simulink model "GEWT_MSC_parthelper2"  (R2015b)
settings: Solver=VariableStepAuto  StartTime=0.0  StopTime=10.0  RelTol=1e-3
values from neighbouring files (symbols this model uses):
  drivefreq = 30e3    (= 30000)    [GEWT.m]
  fluxlinkage = 1.5    [GEWT.m]
  gear = 117.4    [GEWT.m]
  Jtotal = Jgen+Jtur/(gear^2)    (= 1143.20731116)    [GEWT.m]
  Ld = 2.48e-4    (= 0.000248)    [GEWT.m]
  Lq = 2.92e-4    (= 0.000292)    [GEWT.m]
  p = 1.225    [GEWT.m]
  Prated = 2750000    [GEWT.m]
  R = 51.5    [GEWT.m]
  Rs = 0.7305e-3    (= 0.0007305)    [GEWT.m]
  Ts = 2E-6    (= 2e-06)    [GEWT.m]
  windspeed = 10    [GEWT.m]
libraries: powerlib x7, powerlib_meascontrol x5, simulink x3
settings Model: Creator=Eren  LastModifiedBy=Eren

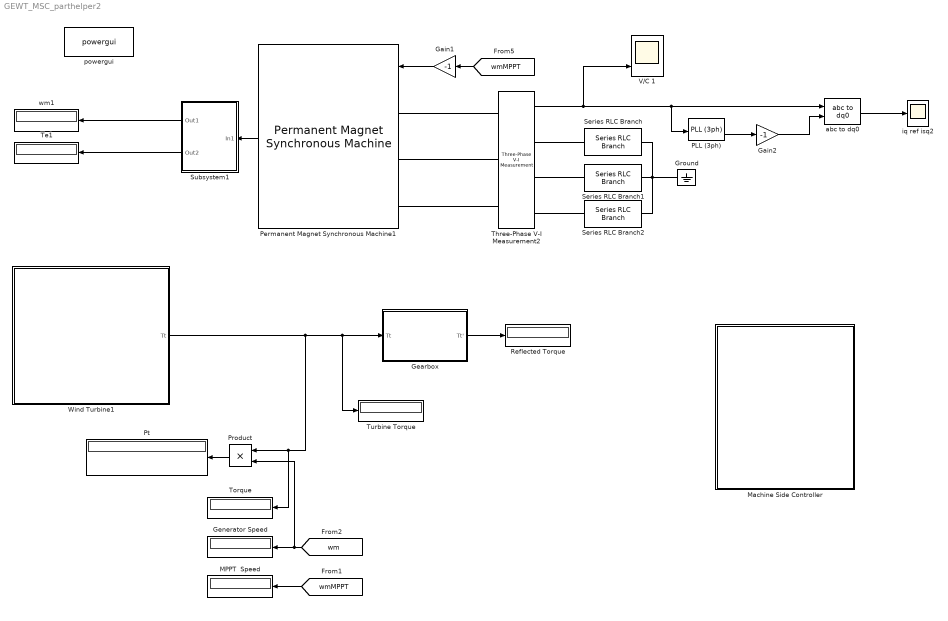
== system GEWT_MSC_parthelper2 ==
  Gain1 : Gain  Gain=-1
  Gain2 : Gain  Gain=-1
  Gearbox : Subsystem
  Generator Speed : Display
  Ground : powerlib/Elements/Ground  LConnTagsString=a
  MPPT  Speed : Display
  "Machine Side Controller " : Subsystem
  PLL (3ph) : powerlib_meascontrol/PLL/PLL (3ph)  Fmin=45  Par_Init=[0, 50]  ParK=[180, 3200, 1]  TcD=1e-4  MaxRateChangeFreq=12  FilterCutOffFreq=25  Ts=Ts  AGC=on
  Permanent Magnet Synchronous Machine1 : powerlib/Machines/Permanent Magnet Synchronous Machine  NbPhases=3  FluxDistribution=Sinusoidal  RotorType=Salient-pole  MechanicalLoad=Speed w  PresetModel=No  ShowDetailedParameters=on  MeasurementBus=off  Resistance=Rs  Inductance=8.5e-3  dqInductances=[Ld,Lq]  La=0.001764  MachineConstant=Voltage Constant (V_peak L-L / krpm)  Flux=1.7933  VoltageCst=650.538  TorqueCst=5.3799  Flat=120  Mechanical=[Jtotal 1.349e-05 4 0]  PolePairs=2  InitialConditions=[-168.8,0, 0,0]  InitialConditions5ph=[0 0 0 0 0 0]  TsPowergui=0  TsBlock=-1  RefAngle=90 degrees behind phase A axis (modified Park)
  Product : Product
  Pt : Display
  Reflected Torque : Display
  Series RLC Branch : powerlib/Elements/Series RLC Branch  LConnTagsString=__new0  RConnTagsString=__new0  BranchType=R  Resistance=1  Inductance=1e-3  SetiL0=off  InitialCurrent=0  Capacitance=1e-6  Setx0=off  InitialVoltage=0  Measurements=None
  Series RLC Branch1 : powerlib/Elements/Series RLC Branch  LConnTagsString=__new0  RConnTagsString=__new0  BranchType=R  Resistance=1  Inductance=1e-3  SetiL0=off  InitialCurrent=0  Capacitance=1e-6  Setx0=off  InitialVoltage=0  Measurements=None
  Series RLC Branch2 : powerlib/Elements/Series RLC Branch  LConnTagsString=__new0  RConnTagsString=__new0  BranchType=R  Resistance=1  Inductance=1e-3  SetiL0=off  InitialCurrent=0  Capacitance=1e-6  Setx0=off  InitialVoltage=0  Measurements=None
  Subsystem1 : Subsystem
  Te1 : Display
  Three-Phase V-I Measurement2 : powerlib/Measurements/Three-Phase V-I Measurement  VoltageMeasurement=phase-to-ground  SetLabelV=off  LabelV=Vsabc  Vpu=off  VpuLL=off  CurrentMeasurement=yes  SetLabelI=on  LabelI=Isabc  Ipu=off  Pbase=10e6  Vbase=690  OutputType=Complex  PhasorSimulation=off  PSBequivalent=0
  Torque : Display
  Turbine Torque : Display
  V/C 1 : Scope  NumInputPorts=2
  Wind Turbine1 : Subsystem
  abc to dq0 : powerlib_meascontrol/Transformations/abc to dq0  Alignment=90 degrees behind phase A axis
  iq ref isq2 : Scope
  powergui : powerlib/powergui  Priority=2  SimulationMode=Discrete  SolverType=Tustin  SampleTime=Ts  frequency=60  SPID=off  DisableSnubberDevices=off  DisableRonSwitches=off  DisableVfSwitches=off  SwTol=0  DisplayEquations=off  Interpol=off  ExternalGateDelay=off  methode=off  Ts=0  FunctionMessages=off  echomessages=off  HookPort=off  EnableUseOfTLC=off  x0status=blocks  frequencyindice=0  Pbase=100e6  ErrMax=1e-4  Iterations=50  UnitsV=kV  UnitsW=MW  buscounter=0  RestoreLinks=warning  ResistiveCurrentMeasurement=off  Frange=[0:2:500]  Ylog=off  Xlog=on  ShowGrid=off  save=off  variable=ZData  structure=0  ZoomFFT=on  StartTime=0.0  cycles=1  DisplayStyle=1  fundamental=60  FreqAxis=off  MaxFrequency=1000  frequencyindicesteady=1  RmsSteady=1  display=off
  wm1 : Display
  wires:
  Permanent Magnet Synchronous Machine1/1 -> Subsystem1/1(In1)
  Subsystem1/1(Out1) -> wm1/1
  Subsystem1/2(Out2) -> Te1/1
  [wmMPPT] -> Gain1/1
  Gain1/1 -> Permanent Magnet Synchronous Machine1/1
  Three-Phase V-I Measurement2/1 -> PLL (3ph)/1, abc to dq0/1, V/C 1/2
  [wm] -> Generator Speed/1, Product/2
  Product/1 -> Pt/1
  Wind Turbine1/1(Tt) -> Turbine Torque/1, Gearbox/1(Tt), Product/1, Torque/1
  Gearbox/1(Tt') -> Reflected Torque/1
  PLL (3ph)/2 -> Gain2/1
  abc to dq0/1 -> iq ref isq2/1
  Gain2/1 -> abc to dq0/2
  [wmMPPT] -> MPPT  Speed/1
  connections:
  Permanent Magnet Synchronous Machine1/LConn2 -- Three-Phase V-I Measurement2/LConn2
  Permanent Magnet Synchronous Machine1/LConn1 -- Three-Phase V-I Measurement2/LConn1
  Permanent Magnet Synchronous Machine1/LConn3 -- Three-Phase V-I Measurement2/LConn3
  Series RLC Branch2/LConn1 -- Three-Phase V-I Measurement2/RConn3
  Series RLC Branch1/LConn1 -- Three-Phase V-I Measurement2/RConn2
  Series RLC Branch/LConn1 -- Three-Phase V-I Measurement2/RConn1
  Series RLC Branch/RConn1 -- Ground/LConn1 -- Series RLC Branch2/RConn1 -- Series RLC Branch1/RConn1

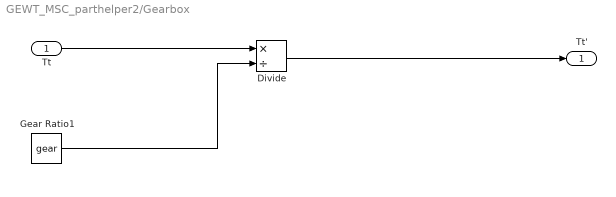
== system GEWT_MSC_parthelper2/Gearbox ==
  Tt : Inport
  Divide : Product  Inputs=*/
  Gear Ratio1 : Constant  Value=gear
  Tt' : Outport
  wires:
  Gear Ratio1/1 -> Divide/2
  Tt/1 -> Divide/1
  Divide/1 -> Tt'/1

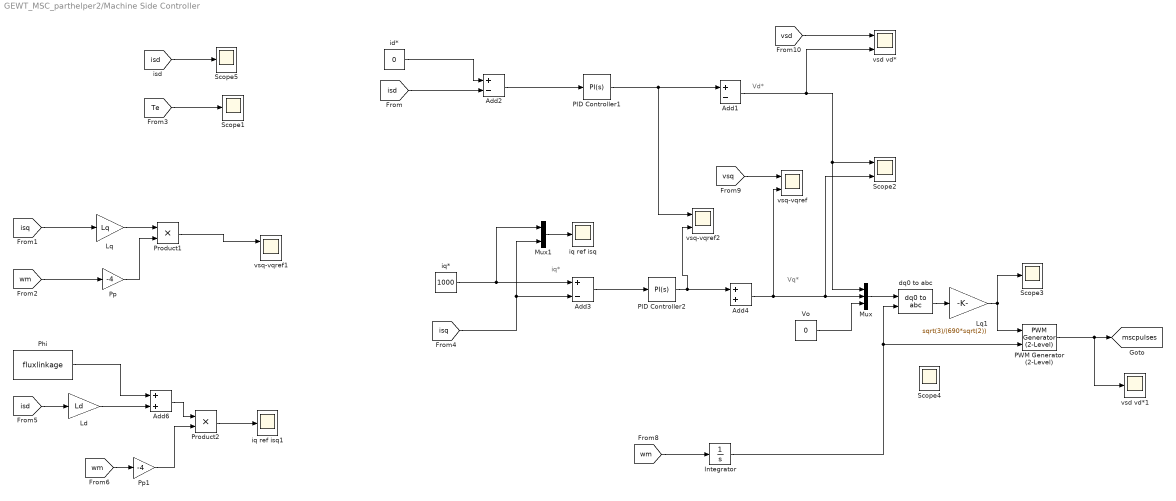
== system GEWT_MSC_parthelper2/Machine Side Controller  ==
  note: iq*
  note: Vq*
  note: Vd*
  Add1 : Sum  Inputs=+-
  Add2 : Sum  Inputs=+-
  Add3 : Sum  Inputs=+-
  Add4 : Sum
  Add6 : Sum
  Integrator : Integrator
  Ld : Gain  Gain=Ld
  Lq : Gain  Gain=Lq
  Lq1 : Gain  Gain=sqrt(3)/(690*sqrt(2))
  Mux : Mux  Inputs=3
  Mux1 : Mux  Inputs=2
  PID Controller1 : simulink/Continuous/PID Controller  Controller=PI  TimeDomain=Continuous-time  SampleTime=-1  IntegratorMethod=Forward Euler  FilterMethod=Forward Euler  Form=Ideal  UseFilter=on  ControllerParametersSource=internal  P=0.0001  I=0.00001  D=0  N=100  InitialConditionSource=internal  InitialConditionForIntegrator=0  InitialConditionForFilter=0  ExternalReset=none  LimitOutput=on  UpperSaturationLimit=2*690  LowerSaturationLimit=-2*690  LinearizeAsGain=on  AntiWindupMode=none  Kb=1  TrackingMode=off  Kt=1  PParamMin=[]  PParamMax=[]  IParamMin=[]  IParamMax=[]  DParamMin=[]  DParamMax=[]  NParamMin=[]  NParamMax=[]  KbParamMin=[]  KbParamMax=[]  KtParamMin=[]  KtParamMax=[]  POutMin=[]  POutMax=[]  IOutMin=[]  IOutMax=[]  DOutMin=[]  DOutMax=[]  NOutMin=[]  NOutMax=[]  KbOutMin=[]  KbOutMax=[]  KtOutMin=[]  KtOutMax=[]  IntegratorOutMin=[]  IntegratorOutMax=[]  FilterOutMin=[]  FilterOutMax=[]  SumOutMin=[]  SumOutMax=[]  SumI1OutMin=[]  SumI1OutMax=[]  SumI2OutMin=[]  SumI2OutMax=[]  SumI3OutMin=[]  SumI3OutMax=[]  SumDOutMin=[]  SumDOutMax=[]  SaturationOutMin=[]  SaturationOutMax=[]  IntegratorContinuousStateAttributes=''  IntegratorStateMustResolveToSignalObject=off  IntegratorRTWStateStorageClass=Auto  FilterContinuousStateAttributes=''  FilterStateMustResolveToSignalObject=off  FilterRTWStateStorageClass=Auto  DifferentiatorICPrevScaledInput=0  DifferentiatorOutMin=[]  DifferentiatorOutMax=[]
  PID Controller2 : simulink/Continuous/PID Controller  Controller=PI  TimeDomain=Continuous-time  SampleTime=-1  IntegratorMethod=Forward Euler  FilterMethod=Forward Euler  Form=Ideal  UseFilter=on  ControllerParametersSource=internal  P=0.0001  I=0.00001  D=0  N=100  InitialConditionSource=internal  InitialConditionForIntegrator=0  InitialConditionForFilter=0  ExternalReset=none  LimitOutput=on  UpperSaturationLimit=2*690  LowerSaturationLimit=-2*690  LinearizeAsGain=on  AntiWindupMode=none  Kb=1  TrackingMode=off  Kt=1  PParamMin=[]  PParamMax=[]  IParamMin=[]  IParamMax=[]  DParamMin=[]  DParamMax=[]  NParamMin=[]  NParamMax=[]  KbParamMin=[]  KbParamMax=[]  KtParamMin=[]  KtParamMax=[]  POutMin=[]  POutMax=[]  IOutMin=[]  IOutMax=[]  DOutMin=[]  DOutMax=[]  NOutMin=[]  NOutMax=[]  KbOutMin=[]  KbOutMax=[]  KtOutMin=[]  KtOutMax=[]  IntegratorOutMin=[]  IntegratorOutMax=[]  FilterOutMin=[]  FilterOutMax=[]  SumOutMin=[]  SumOutMax=[]  SumI1OutMin=[]  SumI1OutMax=[]  SumI2OutMin=[]  SumI2OutMax=[]  SumI3OutMin=[]  SumI3OutMax=[]  SumDOutMin=[]  SumDOutMax=[]  SaturationOutMin=[]  SaturationOutMax=[]  IntegratorContinuousStateAttributes=''  IntegratorStateMustResolveToSignalObject=off  IntegratorRTWStateStorageClass=Auto  FilterContinuousStateAttributes=''  FilterStateMustResolveToSignalObject=off  FilterRTWStateStorageClass=Auto  DifferentiatorICPrevScaledInput=0  DifferentiatorOutMin=[]  DifferentiatorOutMax=[]
  PWM Generator (2-Level) : powerlib_meascontrol/Pulse & Signal Generators/PWM Generator (2-Level)  ModulatorType=Three-phase bridge (6 pulses)  ModulatorMode=Synchronized  Fc=drivefreq  Pc=90  nF=drivefreq/50  MinMax="[ -1  1 ]"  SamplingTechnique=Natural  ModulatingSignals=off  m=0.8  Freq=60  Phase=0  Ts=Ts  ShowCarrierOutport=off
  Phi : Constant  Value=fluxlinkage
  Pp : Gain  Gain=-4
  Pp1 : Gain  Gain=-4
  Product1 : Product
  Product2 : Product
  Scope{1,3..5} (4 alike) : Scope
  Scope2 : Scope  NumInputPorts=2
  Vo : Constant  Value=0
  dq0 to abc : powerlib_meascontrol/Transformations/dq0 to abc  Alignment=90 degrees behind phase A axis
  id* : Constant  Value=0
  iq ref isq : Scope
  iq ref isq1 : Scope
  iq* : Constant  Value=1000
  vsd vd* : Scope  NumInputPorts=2
  vsd vd*1 : Scope
  vsq-vqref : Scope  NumInputPorts=2
  vsq-vqref1 : Scope  NumInputPorts=2
  vsq-vqref2 : Scope  NumInputPorts=2
  tag scope: mscpulses=global
  wires:
  dq0 to abc/1 -> Lq1/1
  Mux/1 -> dq0 to abc/1
  id*/1 -> Add2/1
  Vo/1 -> Mux/3
  [isq] -> Add3/2, Mux1/2
  [wm] -> Pp1/1
  Add3/1 -> PID Controller2/1
  Add2/1 -> PID Controller1/1
  Pp1/1 -> Product2/2
  Ld/1 -> Add6/2
  [isd] -> Add2/2
  Lq/1 -> Product1/1
  Phi/1 -> Add6/1
  PID Controller1/1 -> vsq-vqref2/1, Add1/1
  Add6/1 -> Product2/1
  Pp/1 -> Product1/2
  [isd] -> Ld/1
  [wm] -> Pp/1
  PID Controller2/1 -> vsq-vqref2/2, Add4/1
  [isq] -> Lq/1
  [vsq] -> vsq-vqref/1
  [vsd] -> vsd vd*/1
  Mux1/1 -> iq ref isq/1
  Product1/1 -> vsq-vqref1/1
  [isd] -> Scope5/1
  [Te] -> Scope1/1
  PWM Generator (2-Level)/1 -> [mscpulses], vsd vd*1/1
  Add1/1 -> Scope2/1, Mux/1, vsd vd*/2
  Add4/1 -> Mux/2, Scope2/2, vsq-vqref/2
  iq*/1 -> Add3/1, Mux1/1
  Product2/1 -> iq ref isq1/1
  Lq1/1 -> PWM Generator (2-Level)/1, Scope3/1
  [wm] -> Integrator/1
  Integrator/1 -> PWM Generator (2-Level)/2, dq0 to abc/2

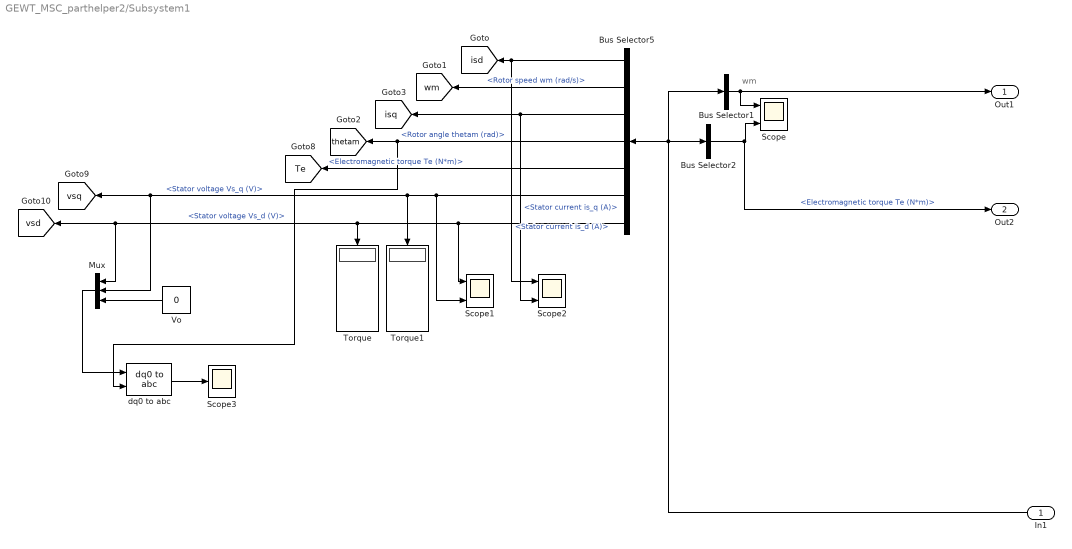
== system GEWT_MSC_parthelper2/Subsystem1 ==
  note: wm
  In1 : Inport
  Bus Selector1 : BusSelector  OutputSignals=Rotor speed wm (rad/s)  OutputAsBus=on
  Bus Selector2 : BusSelector  OutputSignals=Electromagnetic torque Te (N*m)
  Bus Selector5 : BusSelector  OutputSignals=Stator current is_d (A),Rotor speed wm (rad/s),Stator current is_q (A),Rotor angle thetam (rad),Electromagnetic torque Te (N*m),Stator voltage Vs_q (V),Stator voltage Vs_d (V)
  Mux : Mux  Inputs=3
  Scope : Scope  NumInputPorts=2
  Scope1 : Scope  NumInputPorts=2
  Scope2 : Scope  NumInputPorts=2
  Scope3 : Scope
  Torque : Display
  Torque1 : Display
  Vo : Constant  Value=0
  dq0 to abc : powerlib_meascontrol/Transformations/dq0 to abc  Alignment=90 degrees behind phase A axis
  Out1 : Outport
  Out2 : Outport  Port=2
  tag scope: Te=global, isd=global, isq=global, thetam=global, vsd=global, vsq=global, wm=global
  wires:
  Bus Selector1/1 -> Out1/1, Scope/1
  In1/1 -> Bus Selector5/1, Bus Selector1/1, Bus Selector2/1
  Bus Selector5/1 -> Scope2/1, [isd]  "<Stator current is_d (A)>"
  Bus Selector2/1 -> Out2/1, Scope/2  "<Electromagnetic torque Te (N*m)>"
  Bus Selector5/3 -> Scope2/2, [isq]  "<Stator current is_q (A)>"
  Bus Selector5/4 -> dq0 to abc/2, [thetam]  "<Rotor angle thetam (rad)>"
  Bus Selector5/5 -> [Te]  "<Electromagnetic torque Te (N*m)>"
  Bus Selector5/6 -> Scope1/2, Mux/2, [vsq], Torque1/1  "<Stator voltage Vs_q (V)>"
  Bus Selector5/7 -> Scope1/1, Mux/1, [vsd], Torque/1  "<Stator voltage Vs_d (V)>"
  Bus Selector5/2 -> [wm]  "<Rotor speed wm (rad/s)>"
  Vo/1 -> Mux/3
  Mux/1 -> dq0 to abc/1
  dq0 to abc/1 -> Scope3/1

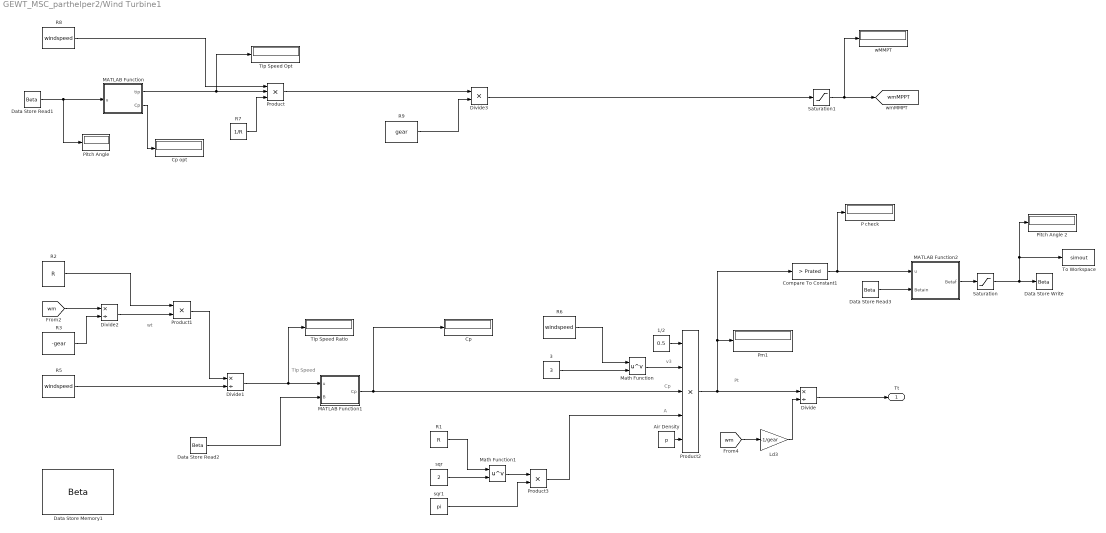
== system GEWT_MSC_parthelper2/Wind Turbine1 ==
  note: Pt
  note: v3
  note: Cp
  note: A
  note: wt
  note: Tip Speed
  1/2 : Constant  Value=0.5
  3 : Constant  Value=3
  Air Density : Constant  Value=p
  Compare To Constant1 : simulink/Logic and Bit Operations/Compare To Constant  relop=>  const=Prated  OutDataTypeStr=boolean
  Cp : Display
  Cp opt : Display
  Data Store Memory1 : DataStoreMemory  DataStoreName=Beta  ReadBeforeWriteMsg=warning  WriteAfterWriteMsg=warning  WriteAfterReadMsg=warning  OutMin=[0]  OutMax=[90]
  Data Store Read1 : DataStoreRead  DataStoreName=Beta  SampleTime=Ts
  Data Store Read2 : DataStoreRead  DataStoreName=Beta  SampleTime=Ts
  Data Store Read3 : DataStoreRead  DataStoreName=Beta  SampleTime=Ts
  Data Store Write : DataStoreWrite  DataStoreName=Beta
  Divide : Product  Inputs=*/
  Divide1 : Product  Inputs=*/
  Divide2 : Product  Inputs=*/
  Divide3 : Product  Inputs=**
  Ld3 : Gain  Gain=-1/gear
  MATLAB Function : MATLAB Function  TreatAsAtomicUnit=on
  MATLAB Function1 : MATLAB Function  TreatAsAtomicUnit=on
  MATLAB Function2 : MATLAB Function  TreatAsAtomicUnit=on
  Math Function : Math  Operator=pow  SaturateOnIntegerOverflow=on
  Math Function1 : Math  Operator=pow  SaturateOnIntegerOverflow=on
  P check : Display
  "Pitch Angle " : Display
  Pitch Angle 2 : Display
  Pm1 : Display
  Product : Product  Inputs=3
  Product1 : Product
  Product2 : Product  Inputs=5
  Product3 : Product
  R1 : Constant  Value=R
  R2 : Constant  Value=R
  R3 : Constant  Value=-gear
  R5 : Constant  Value=windspeed
  R6 : Constant  Value=windspeed
  R7 : Constant  Value=1/R
  R8 : Constant  Value=windspeed
  R9 : Constant  Value=gear
  Saturation : Saturate  UpperLimit=90  LowerLimit=0
  Saturation1 : Saturate  UpperLimit=181.68  LowerLimit=0
  "Tip Speed Opt " : Display
  "Tip Speed Ratio " : Display
  To Workspace : ToWorkspace  VariableName=simout  SaveFormat=Timeseries  SampleTime=-1
  sqr : Constant  Value=2
  sqr1 : Constant  Value=pi
  "wMMPT " : Display
  Tt : Outport
  tag scope: wmMPPT=global
  wires:
  Air Density/1 -> Product2/5
  1/2/1 -> Product2/1
  Product3/1 -> Product2/4
  Math Function1/1 -> Product3/1
  sqr1/1 -> Product3/2
  [wm] -> Ld3/1
  Math Function/1 -> Product2/2
  sqr/1 -> Math Function1/2
  R1/1 -> Math Function1/1
  Divide/1 -> Tt/1
  Product2/1 -> Divide/1, Compare To Constant1/1, Pm1/1
  3/1 -> Math Function/2
  R2/1 -> Product1/1
  [wm] -> Divide2/1
  Product1/1 -> Divide1/1
  R5/1 -> Divide1/2
  Divide1/1 -> MATLAB Function1/1(u), "Tip Speed Ratio "/1
  Divide2/1 -> Product1/2
  Ld3/1 -> Divide/2
  MATLAB Function1/1(Cp) -> Product2/3, Cp/1
  R3/1 -> Divide2/2
  R6/1 -> Math Function/1
  MATLAB Function/1(tip) -> "Tip Speed Opt "/1, Product/2
  R7/1 -> Product/3
  R8/1 -> Product/1
  Product/1 -> Divide3/1
  R9/1 -> Divide3/2
  MATLAB Function/2(Cp) -> Cp opt/1
  Divide3/1 -> Saturation1/1
  Data Store Read3/1 -> MATLAB Function2/2(Betain)
  Data Store Read2/1 -> MATLAB Function1/2(B)
  Data Store Read1/1 -> "Pitch Angle "/1, MATLAB Function/1(u)
  MATLAB Function2/1(Betaf) -> Saturation/1
  Compare To Constant1/1 -> MATLAB Function2/1(u), P check/1
  Saturation/1 -> To Workspace/1, Pitch Angle 2/1, Data Store Write/1
  Saturation1/1 -> "wMMPT "/1, [wmMPPT]

== matlab function GEWT_MSC_parthelper2/Wind Turbine1/MATLAB Function ==
  data: u input; tip output; Cp output
function [tip,Cp]= fcn(u)

c1 = 0.5176;
c2 = 116;
c3 = 0.4;
c4 = 5;
c5 = 21;
c6 = 0.0068;
B=0;
for i = 0.1:0.1:15
    
li = 1/((1/(i+0.08*u))-(0.035/(u^3+1)));
A = c1*((c2/li-c3*u-c4)*exp(-c5/li))+c6*i ;%#codegen

    if A < B
    lopt = i;
    break
    else 
    B = A;
    end
end
tip = i;
Cp = c1*((c2/li-c3*u-c4)*exp(-c5/li))+c6*i;
end

== matlab function GEWT_MSC_parthelper2/Wind Turbine1/MATLAB Function1 ==
  data: u input; B input; Cp output
function Cp = fcn(u,B)

c1 = 0.5176;
c2 = 116;
c3 = 0.4; 
c4 = 5;
c5 = 21;
c6 = 0.0068;

i =u;

li = 1/((1/(i+0.08*B))-(0.035/(B^3+1)));

Cp = c1*((c2/li-c3*B-c4)*exp(-c5/li))+c6*i;

end

== matlab function GEWT_MSC_parthelper2/Wind Turbine1/MATLAB Function2 ==
  data: u input; Betaf output; Betain input
function Betaf  = fcn(u,Betain)

    if u ==1
    Betaf = Betain+0.01;
    else  

    Betaf = Betain-0.01;
    end
 
    
    
end
